simulink library "oneThrSP_cl"  (R2018b)
settings: Solver=VariableStepAuto  StartTime=0.0  StopTime=10.0  RelTol=1e-3
undefined symbols (not defined in the file): rollAmp, startRoll
libraries: threeThrSP_cl x1
settings Model: Creator=asiddiq2  LastModifiedBy=asiddiq2

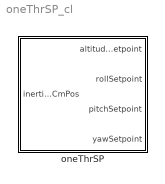
== system oneThrSP_cl ==
  oneThrSP : Subsystem

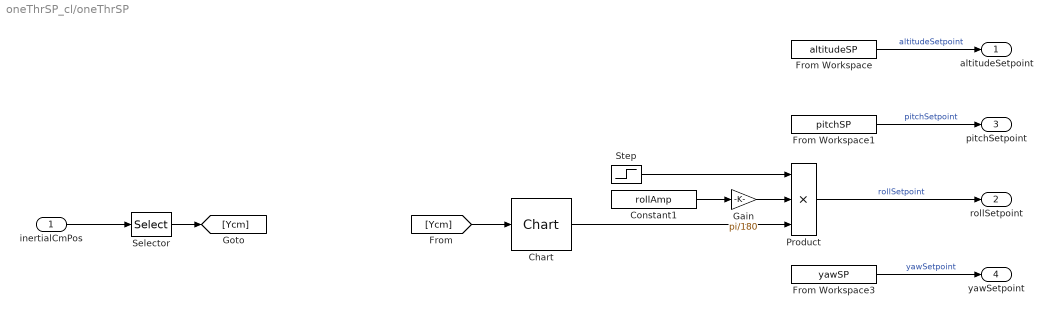
== system oneThrSP_cl/oneThrSP ==
  inertialCmPos : Inport
  Chart : threeThrSP_cl/threeThrSP/Chart  SystemSampleTime=-1
  Constant1 : Constant  Value=rollAmp
  From Workspace : FromWorkspace  VariableName=altitudeSP  SampleTime=0
  From Workspace1 : FromWorkspace  VariableName=pitchSP  SampleTime=0
  From Workspace3 : FromWorkspace  VariableName=yawSP  SampleTime=0
  Gain : Gain  Gain=pi/180
  Product : Product  Inputs=3
  Selector : Selector  InputPortWidth=3  IndexOptions=Index vector (dialog)  Indices=2  OutputSizes=1
  Step : Step  Time=startRoll  SampleTime=0
  altitudeSetpoint : Outport
  rollSetpoint : Outport  Port=2
  pitchSetpoint : Outport  Port=3
  yawSetpoint : Outport  Port=4
  wires:
  Gain/1 -> Product/2
  From Workspace3/1 -> yawSetpoint/1  "yawSetpoint"
  From Workspace1/1 -> pitchSetpoint/1  "pitchSetpoint"
  Constant1/1 -> Gain/1
  From Workspace/1 -> altitudeSetpoint/1  "altitudeSetpoint"
  Chart/1 -> Product/3
  Product/1 -> rollSetpoint/1  "rollSetpoint"
  Selector/1 -> [Ycm]
  inertialCmPos/1 -> Selector/1
  Step/1 -> Product/1
  [Ycm] -> Chart/1
